simulink model "Part2_SimulinkModel"  (R2021a)
settings: Solver=ode23tb  StartTime=0.0  StopTime=90  RelTol=1e-3  EnableMultiTasking=on
libraries: aerolibanim x1, SignalEditorBlockLib x1
settings Model: Creator=Farhan  LastModifiedBy=wadiafa1
settings SolverCC: AlgebraicLoopSolver=TrustRegion
settings DataIOCC: ReturnWorkspaceOutputs=off
settings OptimizationCC: LifeSpan=inf
settings DebuggingCC: SFUnexpectedBacktrackingDiag=warning  SFNoUnconditionalDefaultTransitionDiag=warning  SFMachineParentedDataDiag=warning  ArithmeticOperatorsInVariantConditions=warning
settings SFSimCC: SimUseLocalCustomCode=off  CustomCodeUndefinedFunction=UseInterfaceOnly
settings RTWCC: RTWUseLocalCustomCode=off
settings CodeAppCC: StateflowObjectComments=on
settings GRTTargetCC: TargetLangStandard=C89/C90 (ANSI)
settings ConfigComp: CovMetricSettings=dw  CovSaveCumulativeToWorkspaceVar=on  CovSaveSingleToWorkspaceVar=on  CovExternalEMLEnable=off

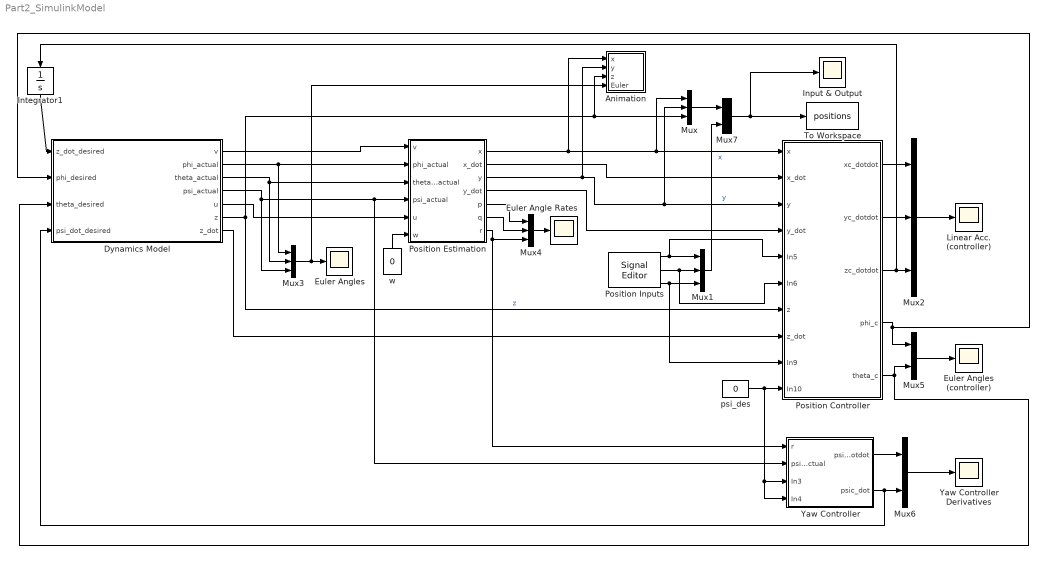
== system Part2_SimulinkModel ==
  Animation : Subsystem
  Dynamics Model : Subsystem
  Euler Angle Rates : Scope
  Euler Angles : Scope
  Euler Angles (controller) : Scope
  Input & Output : Scope
  Integrator1 : Integrator
  Linear Acc. (controller) : Scope
  Mux{,1..4} (5 alike) : Mux  Inputs=3
  Mux5 : Mux  Inputs=2
  Mux6 : Mux  Inputs=2
  Mux7 : Mux  Inputs=2
  Position Controller : Subsystem
  Position Estimation : Subsystem
  Position Inputs : SignalEditorBlockLib/Signal Editor  FileName=input_signals.mat  ActiveScenario=Input  ActiveSignal=x  IsBus=off  OutputBusObjectStr=Bus: BusObject  SampleTime=0  Interpolate=off  ZeroCross=off  OutputAfterFinalValue=Setting to zero  Unit=inherit  PreserveSignalName=on
  To Workspace : ToWorkspace  VariableName=positions  SaveFormat=Structure With Time  SampleTime=-1
  Yaw Controller : Subsystem
  Yaw Controller Derivatives : Scope
  psi_des : Constant  Value=0
  w : Constant  Value=0
  wires:
  Position Estimation/1(x) -> Animation/1(x), Position Controller/1(x), Mux/1  "x"
  Position Estimation/3(y) -> Animation/2(y), Mux/2, Position Controller/3(y)  "y"
  Dynamics Model/6(z) -> Position Controller/7(z), Animation/3(z), Mux/3  "z"
  Position Estimation/2(x_dot) -> Position Controller/2(x_dot)
  Position Estimation/4(y_dot) -> Position Controller/4(y_dot)
  Position Estimation/7(r) -> Yaw Controller/1(r), Mux4/3
  Dynamics Model/5(u) -> Position Estimation/5(u)
  Dynamics Model/4(psi_actual) -> Mux3/3, Yaw Controller/2(psi_actual), Position Estimation/4(psi_actual)
  Dynamics Model/3(theta_actual) -> Mux3/2, Position Estimation/3(theta_actual)
  Dynamics Model/2(phi_actual) -> Position Estimation/2(phi_actual), Mux3/1
  Dynamics Model/1(v) -> Position Estimation/1(v)
  psi_des/1 -> Yaw Controller/4(In4), Yaw Controller/3(In3), Position Controller/10(In10)
  Position Controller/1(xc_dotdot) -> Mux2/1
  Position Controller/2(yc_dotdot) -> Mux2/2
  Position Controller/4(phi_c) -> Dynamics Model/2(phi_desired), Mux5/1
  Position Controller/5(theta_c) -> Dynamics Model/3(theta_desired), Mux5/2
  Yaw Controller/2(psic_dot) -> Mux6/2, Dynamics Model/4(psi_dot_desired)
  w/1 -> Position Estimation/6(w)
  Mux/1 -> Mux7/1
  Position Inputs/1 -> Mux1/1, Position Controller/5(In5)
  Position Inputs/2 -> Position Controller/6(In6), Mux1/2
  Position Inputs/3 -> Position Controller/9(In9), Mux1/3
  Mux1/1 -> Mux7/2
  Position Controller/3(zc_dotdot) -> Mux2/3, Integrator1/1
  Mux2/1 -> Linear Acc. (controller)/1
  Mux3/1 -> Animation/4(Euler), Euler Angles/1
  Position Estimation/5(p) -> Mux4/1
  Position Estimation/6(q) -> Mux4/2
  Mux4/1 -> Euler Angle Rates/1
  Mux5/1 -> Euler Angles (controller)/1
  Yaw Controller/1(psic_dotdot) -> Mux6/1
  Mux6/1 -> Yaw Controller Derivatives/1
  Mux7/1 -> Input & Output/1, To Workspace/1
  Dynamics Model/7(z_dot) -> Position Controller/8(z_dot)
  Integrator1/1 -> Dynamics Model/1(z_dot_desired)

== system Part2_SimulinkModel/Animation ==
  x : Inport
  y : Inport  Port=2
  z : Inport  Port=3
  Euler : Inport  Port=4
  6DoF Animation : aerolibanim/6DoF Animation  u1=[-8 8 -8 8 -8 0]  u2=0.1  u3=2  u4=[0 0 0]  u5=Fixed position  u6=[-80 -40 -70]  u7=10  u8=on
  Gain : Gain  Gain=-1
  Mux8 : Mux  Inputs=3
  wires:
  z/1 -> Gain/1
  Euler/1 -> 6DoF Animation/2
  x/1 -> Mux8/1
  Mux8/1 -> 6DoF Animation/1
  y/1 -> Mux8/2
  Gain/1 -> Mux8/3

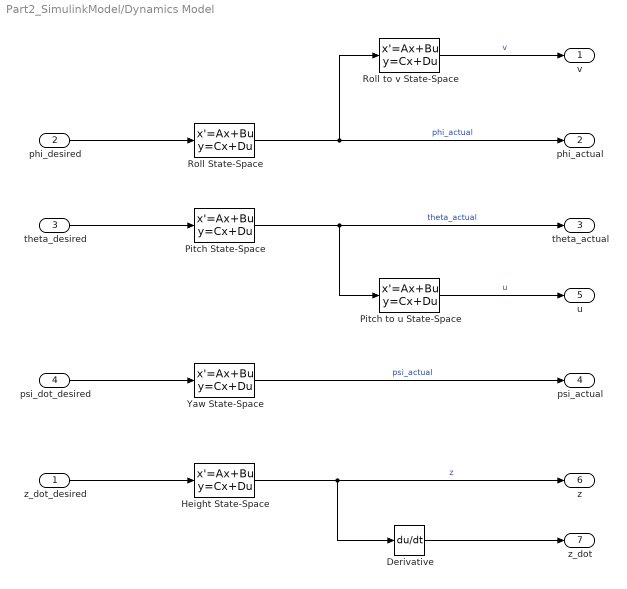
== system Part2_SimulinkModel/Dynamics Model ==
  z_dot_desired : Inport
  phi_desired : Inport  Port=2
  theta_desired : Inport  Port=3
  psi_dot_desired : Inport  Port=4
  Derivative : Derivative
  Height State-Space : StateSpace  A=[-5.82 -3.6046*exp(1)^-6; 3.8147*exp(1)^-6 0]  B=[1024; 0]  C=[1.4907*exp(1)^-4 1.3191*exp(1)^3]  D=0  InitialCondition=0  ContinuousStateAttributes='Height'
  Pitch State-Space : StateSpace  A=[-3.9784 -2.9796; 4 0]  B=[2; 0]  C=[1.2569 0.6083]  D=0  InitialCondition=0  ContinuousStateAttributes='Pitch'
  Pitch to u State-Space : StateSpace  A=-0.665  B=2  C=-3.0772  D=0  InitialCondition=0  ContinuousStateAttributes='Pitch_to_u'
  Roll State-Space : StateSpace  A=[-4.2683 -3.1716; 4 0]  B=[2; 0]  C=[0.7417 0.4405]  D=0  InitialCondition=0  ContinuousStateAttributes='Roll'
  Roll to v State-Space : StateSpace  A=-0.4596  B=2  C=2.3868  D=0  InitialCondition=0  ContinuousStateAttributes='Roll_to_v'
  Yaw State-Space : StateSpace  A=-0.0059  C=1.2653  D=0  InitialCondition=0  ContinuousStateAttributes='Yaw'
  v : Outport
  phi_actual : Outport  Port=2
  theta_actual : Outport  Port=3
  psi_actual : Outport  Port=4
  u : Outport  Port=5
  z : Outport  Port=6
  z_dot : Outport  Port=7
  wires:
  Yaw State-Space/1 -> psi_actual/1  "psi_actual"
  z_dot_desired/1 -> Height State-Space/1
  Height State-Space/1 -> Derivative/1, z/1  "z"
  Roll State-Space/1 -> phi_actual/1, Roll to v State-Space/1  "phi_actual"
  theta_desired/1 -> Pitch State-Space/1
  psi_dot_desired/1 -> Yaw State-Space/1
  Pitch State-Space/1 -> theta_actual/1, Pitch to u State-Space/1  "theta_actual"
  phi_desired/1 -> Roll State-Space/1
  Roll to v State-Space/1 -> v/1  "v"
  Pitch to u State-Space/1 -> u/1  "u"
  Derivative/1 -> z_dot/1

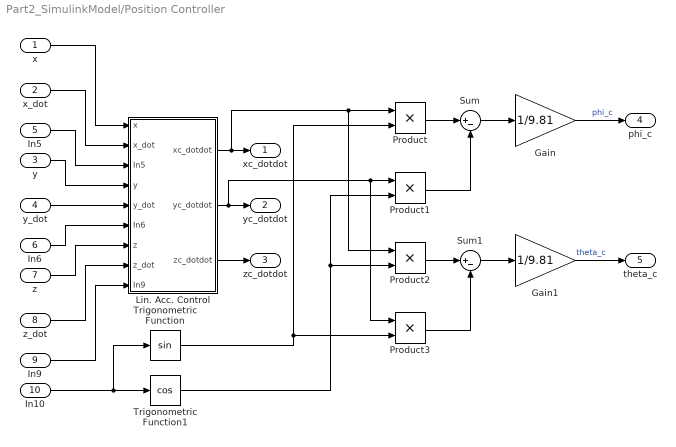
== system Part2_SimulinkModel/Position Controller ==
  x : Inport
  x_dot : Inport  Port=2
  y : Inport  Port=3
  y_dot : Inport  Port=4
  In5 : Inport  Port=5
  In6 : Inport  Port=6
  z : Inport  Port=7
  z_dot : Inport  Port=8
  In9 : Inport  Port=9
  In10 : Inport  Port=10
  Gain : Gain  Gain=1/9.81
  Gain1 : Gain  Gain=1/9.81
  Lin. Acc. Control : Subsystem
  Product{,1..3} (4 alike) : Product
  Sum : Sum  Inputs=|+-
  Sum1 : Sum  Inputs=|+-
  Trigonometric Function : Trigonometry
  Trigonometric Function1 : Trigonometry  Operator=cos
  xc_dotdot : Outport
  yc_dotdot : Outport  Port=2
  zc_dotdot : Outport  Port=3
  phi_c : Outport  Port=4
  theta_c : Outport  Port=5
  wires:
  Lin. Acc. Control/1(xc_dotdot) -> Product2/1, Product/1, xc_dotdot/1
  In5/1 -> Lin. Acc. Control/3(In5)
  y_dot/1 -> Lin. Acc. Control/5(y_dot)
  x_dot/1 -> Lin. Acc. Control/2(x_dot)
  Gain/1 -> phi_c/1  "phi_c"
  Product3/1 -> Sum1/2
  Gain1/1 -> theta_c/1  "theta_c"
  x/1 -> Lin. Acc. Control/1(x)
  z_dot/1 -> Lin. Acc. Control/8(z_dot)
  z/1 -> Lin. Acc. Control/7(z)
  Lin. Acc. Control/3(zc_dotdot) -> zc_dotdot/1
  Trigonometric Function1/1 -> Product1/2, Product2/2
  Product/1 -> Sum/1
  In6/1 -> Lin. Acc. Control/6(In6)
  Sum/1 -> Gain/1
  Product1/1 -> Sum/2
  Product2/1 -> Sum1/1
  In9/1 -> Lin. Acc. Control/9(In9)
  Sum1/1 -> Gain1/1
  y/1 -> Lin. Acc. Control/4(y)
  Lin. Acc. Control/2(yc_dotdot) -> yc_dotdot/1, Product3/1, Product1/1
  Trigonometric Function/1 -> Product/2, Product3/2
  In10/1 -> Trigonometric Function1/1, Trigonometric Function/1

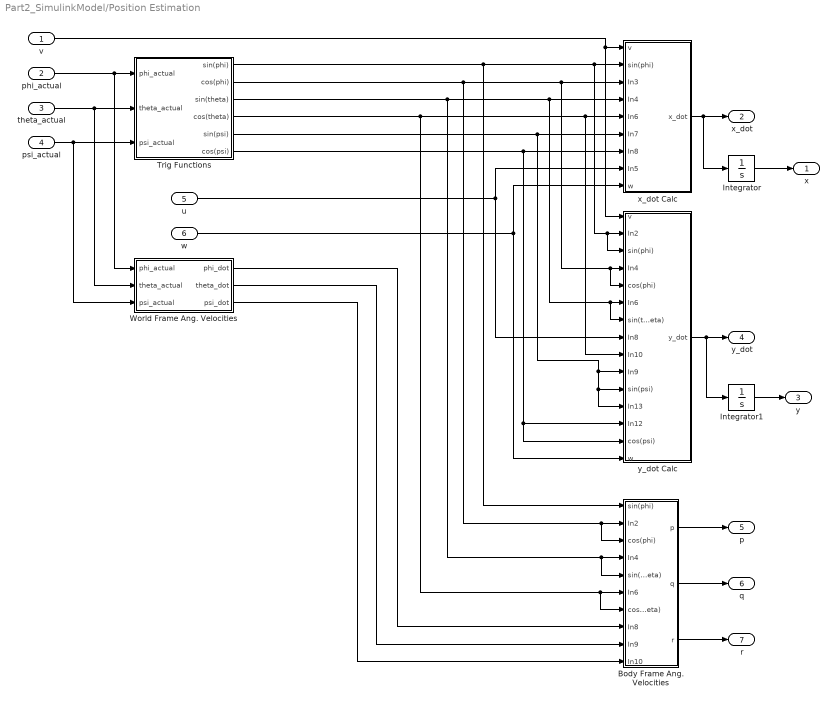
== system Part2_SimulinkModel/Position Estimation ==
  v : Inport
  phi_actual : Inport  Port=2
  theta_actual : Inport  Port=3
  psi_actual : Inport  Port=4
  u : Inport  Port=5
  w : Inport  Port=6
  Body Frame Ang. Velocities : Subsystem
  Integrator : Integrator
  Integrator1 : Integrator
  Trig Functions : Subsystem
  World Frame Ang. Velocities : Subsystem
  x_dot Calc : Subsystem
  y_dot Calc : Subsystem
  x : Outport
  x_dot : Outport  Port=2
  y : Outport  Port=3
  y_dot : Outport  Port=4
  p : Outport  Port=5
  q : Outport  Port=6
  r : Outport  Port=7
  wires:
  Trig Functions/6(cos(psi)) -> y_dot Calc/14(cos(psi)), y_dot Calc/13(In12), x_dot Calc/7(In8)
  w/1 -> x_dot Calc/9(w), y_dot Calc/15(w)
  Body Frame Ang. Velocities/3(r) -> r/1
  Trig Functions/2(cos(phi)) -> y_dot Calc/5(cos(phi)), y_dot Calc/4(In4), x_dot Calc/3(In3), Body Frame Ang. Velocities/3(cos(phi)), Body Frame Ang. Velocities/2(In2)
  Body Frame Ang. Velocities/1(p) -> p/1
  Trig Functions/3(sin(theta)) -> y_dot Calc/7(sin(theta)), y_dot Calc/6(In6), x_dot Calc/4(In4), Body Frame Ang. Velocities/5(sin(theta)), Body Frame Ang. Velocities/4(In4)
  Trig Functions/4(cos(theta)) -> y_dot Calc/9(In10), x_dot Calc/5(In6), Body Frame Ang. Velocities/7(cos(theta)), Body Frame Ang. Velocities/6(In6)
  Trig Functions/5(sin(psi)) -> y_dot Calc/12(In13), y_dot Calc/11(sin(psi)), y_dot Calc/10(In9), x_dot Calc/6(In7)
  y_dot Calc/1(y_dot) -> Integrator1/1, y_dot/1
  u/1 -> x_dot Calc/8(In5), y_dot Calc/8(In8)
  x_dot Calc/1(x_dot) -> Integrator/1, x_dot/1
  World Frame Ang. Velocities/1(phi_dot) -> Body Frame Ang. Velocities/8(In8)
  Body Frame Ang. Velocities/2(q) -> q/1
  World Frame Ang. Velocities/2(theta_dot) -> Body Frame Ang. Velocities/9(In9)
  World Frame Ang. Velocities/3(psi_dot) -> Body Frame Ang. Velocities/10(In10)
  phi_actual/1 -> World Frame Ang. Velocities/1(phi_actual), Trig Functions/1(phi_actual)
  theta_actual/1 -> World Frame Ang. Velocities/2(theta_actual), Trig Functions/2(theta_actual)
  psi_actual/1 -> World Frame Ang. Velocities/3(psi_actual), Trig Functions/3(psi_actual)
  v/1 -> y_dot Calc/1(v), x_dot Calc/1(v)
  Trig Functions/1(sin(phi)) -> Body Frame Ang. Velocities/1(sin(phi)), y_dot Calc/3(sin(phi)), y_dot Calc/2(In2), x_dot Calc/2(sin(phi))
  Integrator/1 -> x/1
  Integrator1/1 -> y/1

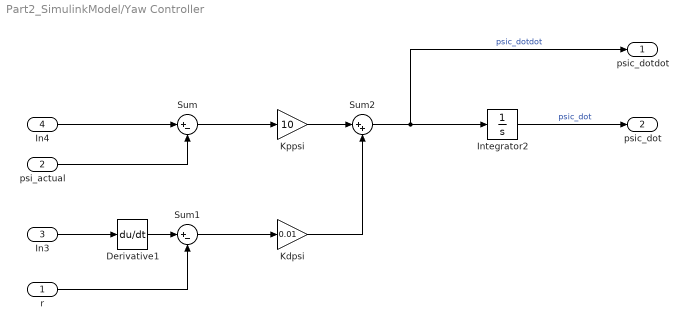
== system Part2_SimulinkModel/Yaw Controller ==
  r : Inport
  psi_actual : Inport  Port=2
  In3 : Inport  Port=3
  In4 : Inport  Port=4
  Derivative1 : Derivative
  Integrator2 : Integrator
  Kdpsi : Gain  Gain=0.01
  Kppsi : Gain  Gain=10
  Sum : Sum  Inputs=|+-
  Sum1 : Sum  Inputs=|+-
  Sum2 : Sum  Inputs=|++
  psic_dotdot : Outport
  psic_dot : Outport  Port=2
  wires:
  Derivative1/1 -> Sum1/1
  Sum1/1 -> Kdpsi/1
  Sum/1 -> Kppsi/1
  Kdpsi/1 -> Sum2/2
  Sum2/1 -> psic_dotdot/1, Integrator2/1  "psic_dotdot"
  In3/1 -> Derivative1/1
  Kppsi/1 -> Sum2/1
  In4/1 -> Sum/1
  r/1 -> Sum1/2
  Integrator2/1 -> psic_dot/1  "psic_dot"
  psi_actual/1 -> Sum/2

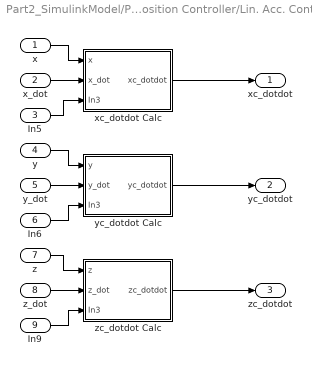
== system Part2_SimulinkModel/Position Controller/Lin. Acc. Control ==
  x : Inport
  x_dot : Inport  Port=2
  In5 : Inport  Port=3
  y : Inport  Port=4
  y_dot : Inport  Port=5
  In6 : Inport  Port=6
  z : Inport  Port=7
  z_dot : Inport  Port=8
  In9 : Inport  Port=9
  xc_dotdot Calc : Subsystem
  yc_dotdot Calc : Subsystem
  zc_dotdot Calc : Subsystem
  xc_dotdot : Outport
  yc_dotdot : Outport  Port=2
  zc_dotdot : Outport  Port=3
  wires:
  xc_dotdot Calc/1(xc_dotdot) -> xc_dotdot/1
  x/1 -> xc_dotdot Calc/1(x)
  yc_dotdot Calc/1(yc_dotdot) -> yc_dotdot/1
  zc_dotdot Calc/1(zc_dotdot) -> zc_dotdot/1
  In9/1 -> zc_dotdot Calc/3(In3)
  In6/1 -> yc_dotdot Calc/3(In3)
  y_dot/1 -> yc_dotdot Calc/2(y_dot)
  z/1 -> zc_dotdot Calc/1(z)
  z_dot/1 -> zc_dotdot Calc/2(z_dot)
  y/1 -> yc_dotdot Calc/1(y)
  In5/1 -> xc_dotdot Calc/3(In3)
  x_dot/1 -> xc_dotdot Calc/2(x_dot)

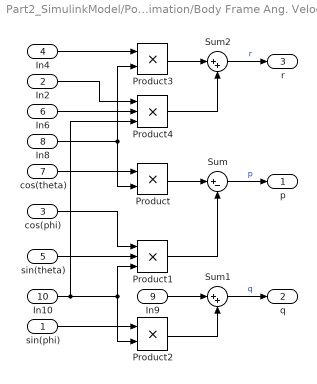
== system Part2_SimulinkModel/Position Estimation/Body Frame Ang. Velocities ==
  sin(phi) : Inport
  In2 : Inport  Port=2
  cos(phi) : Inport  Port=3
  In4 : Inport  Port=4
  sin(theta) : Inport  Port=5
  In6 : Inport  Port=6
  cos(theta) : Inport  Port=7
  In8 : Inport  Port=8
  In9 : Inport  Port=9
  In10 : Inport  Port=10
  Product : Product
  Product1 : Product  Inputs=3
  Product2 : Product
  Product3 : Product
  Product4 : Product  Inputs=3
  Sum : Sum  Inputs=|+-
  Sum1 : Sum  Inputs=|++
  Sum2 : Sum  Inputs=|++
  p : Outport
  q : Outport  Port=2
  r : Outport  Port=3
  wires:
  Product3/1 -> Sum2/1
  Product/1 -> Sum/1
  In9/1 -> Sum1/1
  Sum2/1 -> r/1  "r"
  cos(theta)/1 -> Product/1
  In4/1 -> Product3/1
  Product4/1 -> Sum2/2
  Product1/1 -> Sum/2
  cos(phi)/1 -> Product1/1
  In2/1 -> Product4/1
  sin(theta)/1 -> Product1/2
  Sum1/1 -> q/1  "q"
  Sum/1 -> p/1  "p"
  Product2/1 -> Sum1/2
  In6/1 -> Product4/2
  sin(phi)/1 -> Product2/1
  In10/1 -> Product2/2, Product1/3, Product4/3
  In8/1 -> Product3/2, Product/2

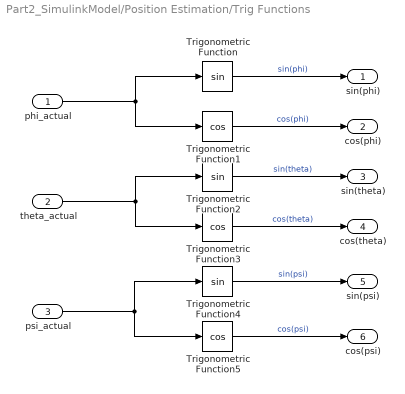
== system Part2_SimulinkModel/Position Estimation/Trig Functions ==
  phi_actual : Inport
  theta_actual : Inport  Port=2
  psi_actual : Inport  Port=3
  Trigonometric Function : Trigonometry
  Trigonometric Function1 : Trigonometry  Operator=cos
  Trigonometric Function2 : Trigonometry
  Trigonometric Function3 : Trigonometry  Operator=cos
  Trigonometric Function4 : Trigonometry
  Trigonometric Function5 : Trigonometry  Operator=cos
  sin(phi) : Outport
  cos(phi) : Outport  Port=2
  sin(theta) : Outport  Port=3
  cos(theta) : Outport  Port=4
  sin(psi) : Outport  Port=5
  cos(psi) : Outport  Port=6
  wires:
  phi_actual/1 -> Trigonometric Function1/1, Trigonometric Function/1
  Trigonometric Function2/1 -> sin(theta)/1  "sin(theta)"
  theta_actual/1 -> Trigonometric Function3/1, Trigonometric Function2/1
  Trigonometric Function1/1 -> cos(phi)/1  "cos(phi)"
  psi_actual/1 -> Trigonometric Function4/1, Trigonometric Function5/1
  Trigonometric Function4/1 -> sin(psi)/1  "sin(psi)"
  Trigonometric Function/1 -> sin(phi)/1  "sin(phi)"
  Trigonometric Function3/1 -> cos(theta)/1  "cos(theta)"
  Trigonometric Function5/1 -> cos(psi)/1  "cos(psi)"

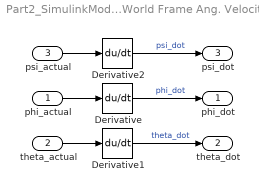
== system Part2_SimulinkModel/Position Estimation/World Frame Ang. Velocities ==
  phi_actual : Inport
  theta_actual : Inport  Port=2
  psi_actual : Inport  Port=3
  Derivative : Derivative
  Derivative1 : Derivative
  Derivative2 : Derivative
  phi_dot : Outport
  theta_dot : Outport  Port=2
  psi_dot : Outport  Port=3
  wires:
  psi_actual/1 -> Derivative2/1
  Derivative/1 -> phi_dot/1  "phi_dot"
  Derivative1/1 -> theta_dot/1  "theta_dot"
  theta_actual/1 -> Derivative1/1
  Derivative2/1 -> psi_dot/1  "psi_dot"
  phi_actual/1 -> Derivative/1

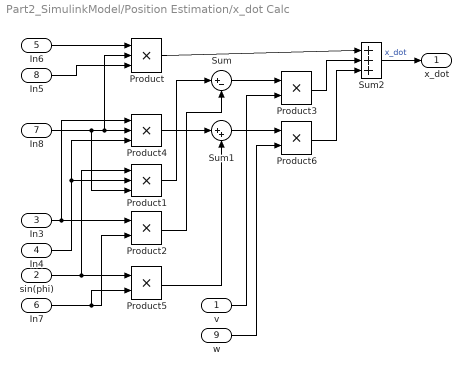
== system Part2_SimulinkModel/Position Estimation/x_dot Calc ==
  v : Inport
  sin(phi) : Inport  Port=2
  In3 : Inport  Port=3
  In4 : Inport  Port=4
  In6 : Inport  Port=5
  In7 : Inport  Port=6
  In8 : Inport  Port=7
  In5 : Inport  Port=8
  w : Inport  Port=9
  Product : Product  Inputs=3
  Product1 : Product  Inputs=3
  Product{2..3,5..6} (4 alike) : Product
  Product4 : Product  Inputs=3
  Sum : Sum  Inputs=|+-
  Sum1 : Sum  Inputs=|++
  Sum2 : Sum  Inputs=|+++
  x_dot : Outport
  wires:
  w/1 -> Product6/2
  Product5/1 -> Sum1/2
  Sum2/1 -> x_dot/1  "x_dot"
  Product/1 -> Sum2/1
  Product1/1 -> Sum/1
  sin(phi)/1 -> Product1/1, Product5/1
  v/1 -> Product3/2
  In8/1 -> Product/2, Product4/2, Product1/3
  Product2/1 -> Sum/2
  Sum/1 -> Product3/1
  Product3/1 -> Sum2/2
  In3/1 -> Product4/1, Product2/1
  In6/1 -> Product/1
  In5/1 -> Product/3
  Sum1/1 -> Product6/1
  Product6/1 -> Sum2/3
  Product4/1 -> Sum1/1
  In7/1 -> Product5/2, Product2/2
  In4/1 -> Product4/3, Product1/2

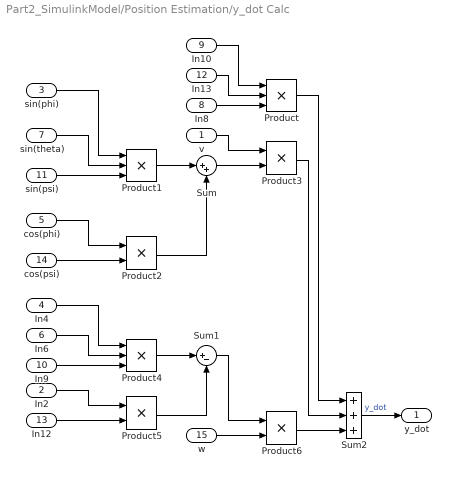
== system Part2_SimulinkModel/Position Estimation/y_dot Calc ==
  v : Inport
  In2 : Inport  Port=2
  sin(phi) : Inport  Port=3
  In4 : Inport  Port=4
  cos(phi) : Inport  Port=5
  In6 : Inport  Port=6
  sin(theta) : Inport  Port=7
  In8 : Inport  Port=8
  In10 : Inport  Port=9
  In9 : Inport  Port=10
  sin(psi) : Inport  Port=11
  In13 : Inport  Port=12
  In12 : Inport  Port=13
  cos(psi) : Inport  Port=14
  w : Inport  Port=15
  Product : Product  Inputs=3
  Product1 : Product  Inputs=3
  Product{2..3,5..6} (4 alike) : Product
  Product4 : Product  Inputs=3
  Sum : Sum  Inputs=|++
  Sum1 : Sum  Inputs=|+-
  Sum2 : Sum  Inputs=+++
  y_dot : Outport
  wires:
  In8/1 -> Product/3
  In12/1 -> Product5/2
  Sum1/1 -> Product6/1
  Product3/1 -> Sum2/2
  In9/1 -> Product4/3
  Product1/1 -> Sum/1
  In2/1 -> Product5/1
  sin(psi)/1 -> Product1/3
  Sum2/1 -> y_dot/1  "y_dot"
  In4/1 -> Product4/1
  Product2/1 -> Sum/2
  w/1 -> Product6/2
  v/1 -> Product3/1
  Product/1 -> Sum2/1
  In13/1 -> Product/2
  In10/1 -> Product/1
  Product6/1 -> Sum2/3
  cos(phi)/1 -> Product2/1
  Product4/1 -> Sum1/1
  sin(theta)/1 -> Product1/2
  Product5/1 -> Sum1/2
  sin(phi)/1 -> Product1/1
  In6/1 -> Product4/2
  cos(psi)/1 -> Product2/2
  Sum/1 -> Product3/2

== system Part2_SimulinkModel/Position Controller/Lin. Acc. Control/xc_dotdot Calc ==
  x : Inport
  x_dot : Inport  Port=2
  In3 : Inport  Port=3
  Kdx : Gain  Gain=35
  Kpx : Gain  Gain=20
  Sum : Sum  Inputs=|+-
  Sum1 : Sum  Inputs=|+-
  xc_dotdot : Outport
  wires:
  Sum/1 -> Kpx/1
  x_dot/1 -> Kdx/1
  Kdx/1 -> Sum1/2
  x/1 -> Sum/2
  In3/1 -> Sum/1
  Sum1/1 -> xc_dotdot/1  "xc_dotdot"
  Kpx/1 -> Sum1/1

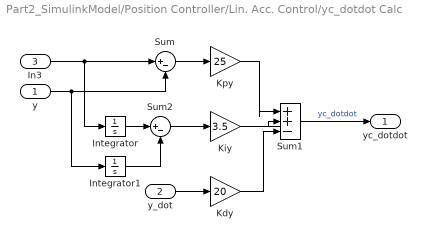
== system Part2_SimulinkModel/Position Controller/Lin. Acc. Control/yc_dotdot Calc ==
  y : Inport
  y_dot : Inport  Port=2
  In3 : Inport  Port=3
  Integrator : Integrator
  Integrator1 : Integrator
  Kdy : Gain  Gain=20
  Kiy : Gain  Gain=3.5
  Kpy : Gain  Gain=25
  Sum : Sum  Inputs=|+-
  Sum1 : Sum  Inputs=|++-
  Sum2 : Sum  Inputs=|+-
  yc_dotdot : Outport
  wires:
  Sum1/1 -> yc_dotdot/1  "yc_dotdot"
  y_dot/1 -> Kdy/1
  Sum/1 -> Kpy/1
  y/1 -> Integrator1/1, Sum/2
  Kpy/1 -> Sum1/1
  In3/1 -> Integrator/1, Sum/1
  Kdy/1 -> Sum1/3
  Integrator/1 -> Sum2/1
  Integrator1/1 -> Sum2/2
  Sum2/1 -> Kiy/1
  Kiy/1 -> Sum1/2

== system Part2_SimulinkModel/Position Controller/Lin. Acc. Control/zc_dotdot Calc ==
  z : Inport
  z_dot : Inport  Port=2
  In3 : Inport  Port=3
  Kdz : Gain  Gain=8
  Kpz : Gain  Gain=30
  Sum : Sum  Inputs=|+-
  Sum1 : Sum  Inputs=|+-
  zc_dotdot : Outport
  wires:
  Kdz/1 -> Sum1/2
  Sum1/1 -> zc_dotdot/1  "zc_dotdot"
  z_dot/1 -> Kdz/1
  Sum/1 -> Kpz/1
  z/1 -> Sum/2
  Kpz/1 -> Sum1/1
  In3/1 -> Sum/1
